simulink model "H8_EMS_comparacionNL_Lineal"  (R2022b)
settings: Solver=VariableStepAuto  StartTime=0.0  StopTime=0.1  RelTol=1e-3
values from neighbouring files (symbols this model uses):
  A1 = [0 0 0 0 0 0 0 0 1 0 0 0 ... (16 elements, 4x4)]    [matrices_linealizacion_ems.mat]
  B1 = [0 0 0.0235189285717 0.0718484523046 0 0 -0.0235189285717 -0.0718484523046 0 0 0.0235189285717 -0.087743417172 ... (16 elements, 4x4)]    [matrices_linealizacion_ems.mat]
  C1 = [1 0 0 0 0 1 0 0 0 0 1 0 ... (16 elements, 4x4)]    [matrices_linealizacion_ems.mat]
  D1 = [0 0 0 0 0 0 0 0 0 0 0 0 ... (16 elements, 4x4)]    [matrices_linealizacion_ems.mat]
settings Model: Creator=USUARIO  LastModifiedBy=USUARIO

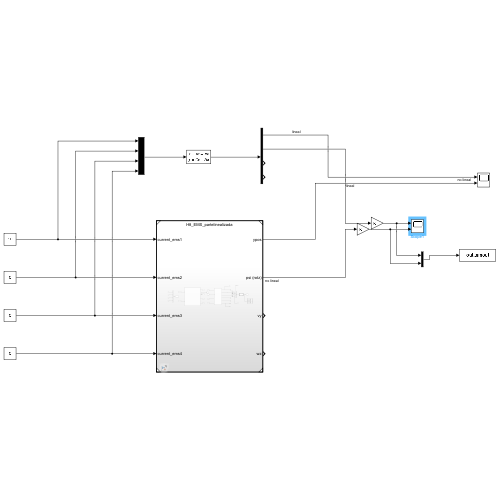
[thumbnail: Simulink's stored preview of the top-level diagram]
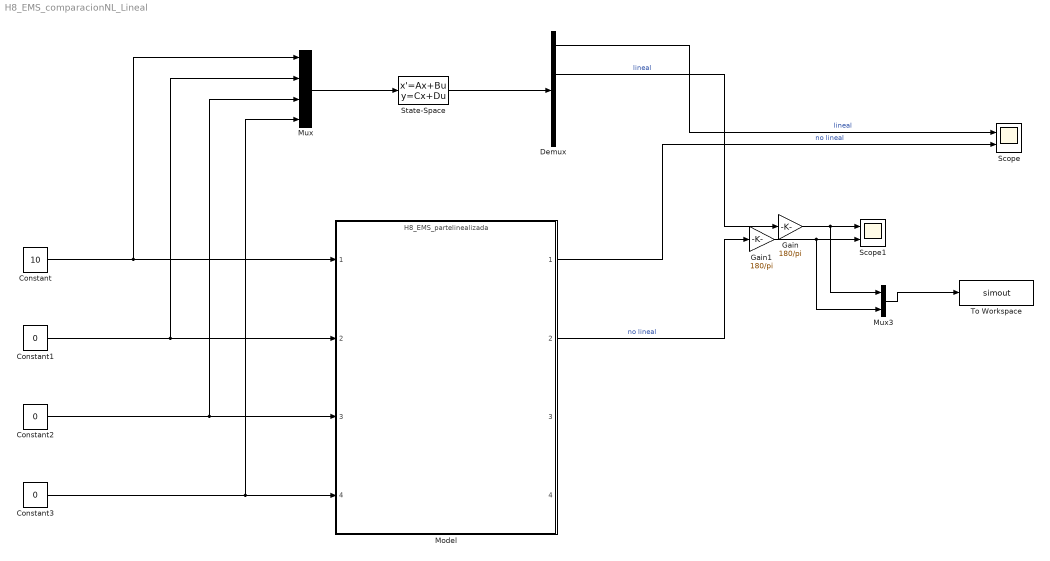
== system H8_EMS_comparacionNL_Lineal ==
  Constant : Constant  Value=10
  Constant1 : Constant  Value=0
  Constant2 : Constant  Value=0
  Constant3 : Constant  Value=0
  Demux : Demux
  Gain : Gain  Gain=180/pi
  Gain1 : Gain  Gain=180/pi
  Model : ModelReference  ModelNameDialog=H8_EMS_partelinealizada.slx  SimulationMode=Normal  ModelReferenceVersion=1.7
  Mux : Mux
  Mux3 : Mux  Inputs=2
  Scope : Scope  NumInputPorts=2
  Scope1 : Scope  NumInputPorts=2
  State-Space : StateSpace  A=A1  B=B1  C=C1  D=D1  InitialCondition=[0.000 , 0.0 , 0, 0.00]
  To Workspace : ToWorkspace  VariableName=simout  SaveFormat=Timeseries  SampleTime=-1
  wires:
  Mux/1 -> State-Space/1
  Demux/1 -> Scope/1  "lineal"
  State-Space/1 -> Demux/1
  Model/1 -> Scope/2  "no lineal"
  Constant2/1 -> Model/3, Mux/3
  Constant1/1 -> Model/2, Mux/2
  Constant3/1 -> Model/4, Mux/4
  Constant/1 -> Model/1, Mux/1
  Model/2 -> Gain1/1  "no lineal"
  Demux/2 -> Gain/1  "lineal"
  Mux3/1 -> To Workspace/1
  Gain1/1 -> Mux3/2, Scope1/2
  Gain/1 -> Mux3/1, Scope1/1
